simulink model "practica7"  (R2023a)
settings: Solver=VariableStepAuto  StartTime=0.0  StopTime=10  RelTol=1e-3
libraries: simulink x2
settings Model: Creator=Juanincho  LastModifiedBy=Juanincho

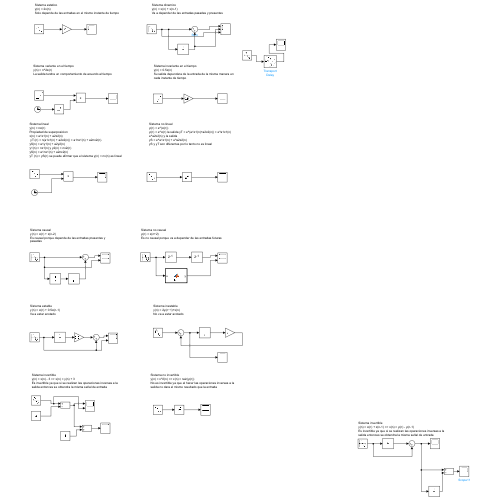
[thumbnail: Simulink's stored preview of the top-level diagram]
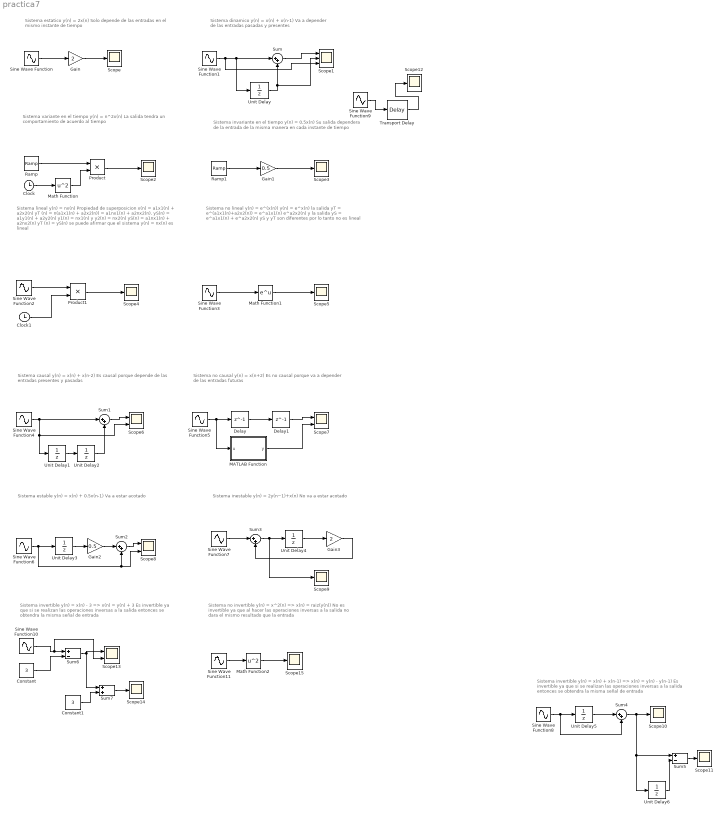
== system practica7 ==
  note: Sistema estatico
      | y(n) = 2x(n)
      | Solo depende de las entradas en el mismo instante de tiempo
  note: Sistema dinamico
      | y(n) = x(n) + x(n-1)
      | Va a depender de las entradas pasadas y presentes
  note: Sistema variante en el tiempo
      | y(n) = n^2x(n)
      | La salida tendra un comportamiento de acuerdo al tiempo
  note: Sistema invariante en el tiempo
      | y(n) = 0.5x(n)
      | Su salida dependera de la entrada de la misma manera en cada instante de tiempo
  note: Sistema lineal
      | y(n) = nx(n)
      | Propiedad de superposicion
      | x(n) = a1x1(n) + a2x2(n)
      | yT (n) = n(a1x1(n) + a2x2(n)) = a1nx1(n) + a2nx2(n).
      | yS(n) = a1y1(n) + a2y2(n)
      | y1(n) = nx1(n) y y2(n) = nx2(n)
      | yS(n) = a1nx1(n) + a2nx2(n)
      | yT (n) = yS(n) se puede afirmar que el sistema y(n) = nx(n) es lineal
  note: Sistema no lineal
      | y(n) = e^(x(n))
      | y(n) = e^x(n) la salida yT = e^(a1x1(n)+a2x2(n)) = e^a1x1(n) e^a2x2(n) y la salida
      | yS = e^a1x1(n) + e^a2x2(n)
      | yS y yT son diferentes por lo tanto no es lineal
  note: Sistema causal
      | y(n) = x(n) + x(n-2)
      | Es causal porque depende de las entradas presentes y pasadas
  note: Sistema no causal
      | y(n) = x(n+2)
      | Es no causal porque va a depender de las entradas futuras
  note: Sistema estable
      | y(n) = x(n) + 0.5x(n-1)
      | Va a estar acotado
  note: Sistema inestable
      | y(n) = 2y(n−1)+x(n)
      | No va a estar acotado
  note: Sistema invertible
      | y(n) = x(n) + x(n-1) => x(n) = y(n) - y(n-1)
      | Es invertible ya que si se realizan las operaciones inversas a la salida entonces se obtendra la misma señal de entrada
  note: Sistema invertible
      | y(n) = x(n) - 3 => x(n) = y(n) + 3
      | Es invertible ya que si se realizan las operaciones inversas a la salida entonces se obtendra la misma señal de entrada
  note: Sistema no invertible
      | y(n) = x^2(n) => x(n) = raiz(y(n))
      | No es invertible ya que al hacer las operaciones inversas a la salida no dara el mismo resultado que la entrada
  Clock : Clock
  Clock1 : Clock
  Constant : Constant  Value=3
  Constant1 : Constant  Value=3
  Delay : Delay  DelayLength=1  InitialCondition=0
  Delay1 : Delay  DelayLength=1  InitialCondition=0
  Gain : Gain  Gain=2
  Gain1 : Gain  Gain=0.5
  Gain2 : Gain  Gain=0.5
  Gain3 : Gain  Gain=2
  MATLAB Function : MATLAB Function  TreatAsAtomicUnit=on
  Math Function : Math  Operator=square
  Math Function1 : Math
  Math Function2 : Math  Operator=square
  Product : Product
  Product1 : Product
  Ramp : simulink/Sources/Ramp  slope=1  start=0  InitialOutput=0
  Ramp1 : simulink/Sources/Ramp  slope=1  start=0  InitialOutput=0
  Scope{,2..5,9..12,14..15} (11 alike) : Scope
  Scope1 : Scope  NumInputPorts=3
  Scope{6..8,13} (4 alike) : Scope  NumInputPorts=2
  Sine Wave Function{,2..3,8,10..11} (6 alike) : Sin  SampleTime=0
  Sine Wave Function{1,4,6..7,9} (5 alike) : Sin  SampleTime=0.2
  Sine Wave Function5 : Sin  SampleTime=0.1
  Sum{,1..4} (5 alike) : Sum  Inputs=|++
  Sum5 : Sum  Inputs=+-
  Sum6 : Sum  Inputs=+-
  Sum7 : Sum
  Transport Delay : TransportDelay
  Unit Delay{,1..6} (7 alike) : UnitDelay  SampleTime=-1  HasFrameUpgradeWarning=on
  wires:
  Sine Wave Function/1 -> Gain/1
  Gain/1 -> Scope/1
  Sine Wave Function1/1 -> Scope1/3, Unit Delay/1, Sum/1
  Sum/1 -> Scope1/1
  Unit Delay/1 -> Scope1/2, Sum/2
  Math Function/1 -> Product/2
  Clock/1 -> Math Function/1
  Product/1 -> Scope2/1
  Ramp/1 -> Product/1
  Ramp1/1 -> Gain1/1
  Gain1/1 -> Scope3/1
  Sine Wave Function2/1 -> Product1/1
  Clock1/1 -> Product1/2
  Product1/1 -> Scope4/1
  Sine Wave Function3/1 -> Math Function1/1
  Math Function1/1 -> Scope5/1
  Sine Wave Function4/1 -> Scope6/2, Unit Delay1/1, Sum1/1
  Unit Delay1/1 -> Unit Delay2/1
  Unit Delay2/1 -> Sum1/2
  Sum1/1 -> Scope6/1
  Delay/1 -> Delay1/1
  Sine Wave Function5/1 -> MATLAB Function/1(u), Delay/1
  Delay1/1 -> Scope7/1
  Sine Wave Function6/1 -> Scope8/2, Sum2/2, Unit Delay3/1
  Unit Delay3/1 -> Gain2/1
  Gain2/1 -> Sum2/1
  Sum2/1 -> Scope8/1
  Sine Wave Function7/1 -> Sum3/1
  Sum3/1 -> Scope9/1, Unit Delay4/1
  Unit Delay4/1 -> Gain3/1
  Gain3/1 -> Sum3/2
  Sine Wave Function8/1 -> Sum4/2, Unit Delay5/1
  Unit Delay5/1 -> Sum4/1
  Sum4/1 -> Unit Delay6/1, Sum5/1, Scope10/1
  Sum5/1 -> Scope11/1
  Unit Delay6/1 -> Sum5/2
  Sine Wave Function10/1 -> Scope13/2, Sum6/1
  Constant/1 -> Sum6/2
  Sum6/1 -> Sum7/1, Scope13/1
  Constant1/1 -> Sum7/2
  Sum7/1 -> Scope14/1
  Sine Wave Function11/1 -> Math Function2/1
  Math Function2/1 -> Scope15/1
  Sine Wave Function9/1 -> Transport Delay/1
  Transport Delay/1 -> Scope12/1
  MATLAB Function/1(y) -> Scope7/2

== matlab function practica7/MATLAB Function ==
  data: u input; y output
function y = fcn(u)

    y = u;
end
